simulink model "test"  (Simulink 8.3)
settings: Solver=ode45  StartTime=0.0  StopTime=100  RelTol=1e-3
values from neighbouring files (symbols this model uses):
  Fa = mdot(v,j)    [Build_sim.m]    (also in opt_build.m = mdot(i,j))
  Fw = water_flow(v+1,j)    [Build_sim.m]    (also in opt_build.m = water_flow(i+1,j))
  tai = SAT_AC(v+1)    [Build_sim.m]    (also in opt_build.m = SAT_iter(i,j))
  twi = 120    [Build_sim.m]    (also in opt_build.m)
settings Model: Creator=meisu  LastModifiedBy=meisu
settings DataIOCC: SignalLoggingSaveFormat=Dataset
settings DebuggingCC: UnderspecifiedInitializationDetection=Simplified  StateNameClashWarn=none
settings GRTTargetCC: CombineOutputUpdateFcns=on  GRTInterface=off

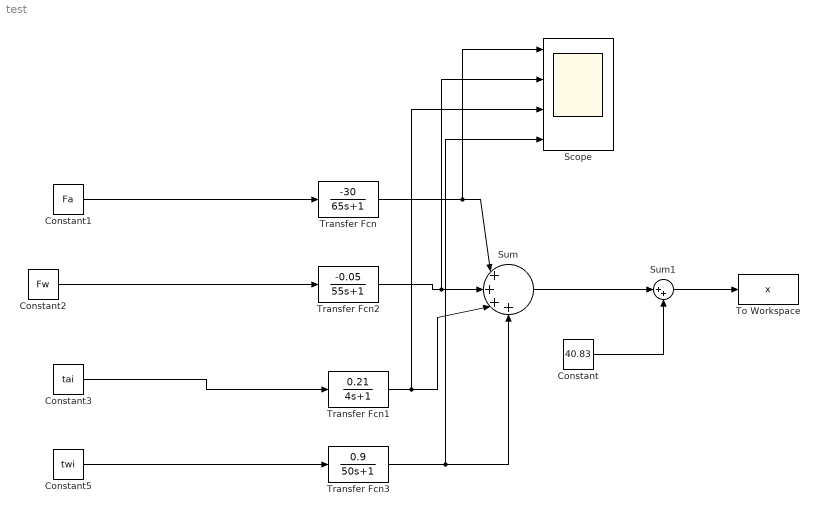
== system test ==
  Constant : Constant  Value=40.83
  Constant1 : Constant  Value=Fa
  Constant2 : Constant  Value=Fw
  Constant3 : Constant  Value=tai
  Constant5 : Constant  Value=twi
  Scope : Scope  NumInputPorts=4
      settings: YMin=-5~-5~-5~-5  YMax=5~5~5~5
  Sum : Sum  Inputs=|++++
  Sum1 : Sum  Inputs=|++
  To Workspace : ToWorkspace  VariableName=x  SaveFormat=Timeseries  SampleTime=-1
  Transfer Fcn : TransferFcn  Numerator=[-30]  Denominator=[65 1]
  Transfer Fcn1 : TransferFcn  Numerator=[0.21]  Denominator=[4 1]
  Transfer Fcn2 : TransferFcn  Numerator=[-0.05]  Denominator=[55 1]
  Transfer Fcn3 : TransferFcn  Numerator=[0.9]  Denominator=[50 1]
  wires:
  Constant1/1 -> Transfer Fcn/1
  Constant5/1 -> Transfer Fcn3/1
  Constant3/1 -> Transfer Fcn1/1
  Constant2/1 -> Transfer Fcn2/1
  Transfer Fcn/1 -> Scope/1, Sum/1
  Transfer Fcn2/1 -> Scope/2, Sum/2
  Transfer Fcn1/1 -> Scope/3, Sum/3
  Transfer Fcn3/1 -> Scope/4, Sum/4
  Constant/1 -> Sum1/2
  Sum/1 -> Sum1/1
  Sum1/1 -> To Workspace/1
